simulink model "task8a_winkel"  (R2024a)
settings: Solver=VariableStepAuto  StartTime=0.0  StopTime=1.5  RelTol=1e-3
libraries: robotmaniplib x1, robotcorelib x1
settings Model: Creator=Nico  LastModifiedBy=laith
settings RTWCC: GPUComputeCapability=3.5

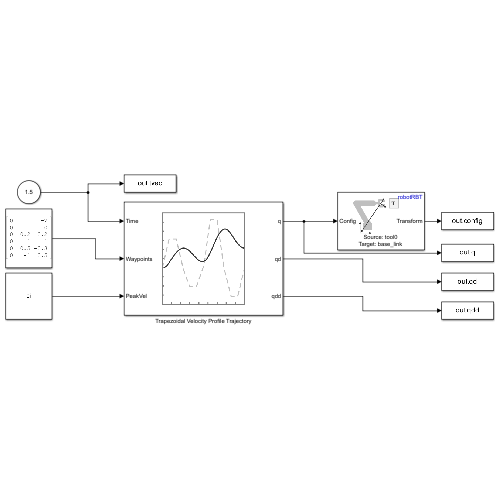
[thumbnail: Simulink's stored preview of the top-level diagram]
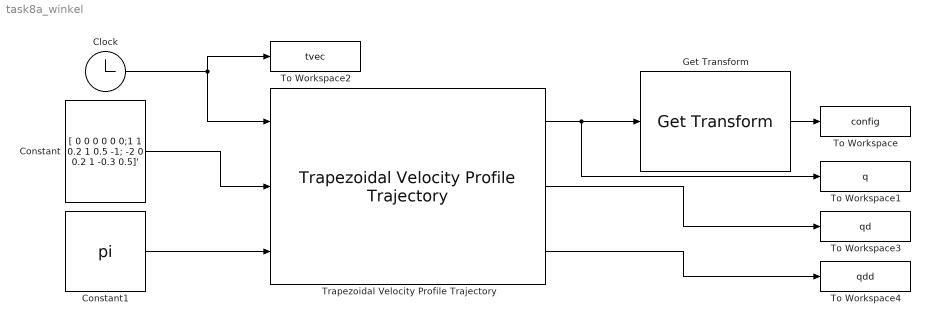
== system task8a_winkel ==
  Clock : Clock
      settings: Decimation=100
  Constant : Constant  Value="[ 0 0 0 0 0 0;1   1  0.2   1    0.5     -1;  -2  0  0.2   1 -0.3    0.5]'"
  Constant1 : Constant  Value=pi
  Get Transform : robotmaniplib/Get Transform  RigidBodyTree=robotRBT  SourceBody=tool0  TargetBody=base_link  SimulateUsing=Interpreted execution
  To Workspace : ToWorkspace  VariableName=config  SampleTime=-1
  To Workspace1 : ToWorkspace  VariableName=q  SampleTime=-1
      settings: Save2DSignal=2-D array (concatenate along first dimension)
  To Workspace2 : ToWorkspace  VariableName=tvec  SampleTime=-1
  To Workspace3 : ToWorkspace  VariableName=qd  SampleTime=-1
      settings: Save2DSignal=2-D array (concatenate along first dimension)
  To Workspace4 : ToWorkspace  VariableName=qdd  SampleTime=-1
      settings: Save2DSignal=2-D array (concatenate along first dimension)
  Trapezoidal Velocity Profile Trajectory : robotcorelib/Trapezoidal Velocity Profile Trajectory  WaypointSource=External  Waypoints=[ 0, -0.5, -1; 0, 0.5, 1 ]  NumParams=1  Parameter1=Peak Velocity  Parameter2=Acceleration  ParameterSource=External  PeakVelocity=[ 2; 2 ]  Acceleration=[ 1; 2 ]  EndTime=[ 1; 1 ]  AccelTime=[ 1; 2 ]  SimulateUsing=Interpreted execution
  wires:
  Constant/1 -> Trapezoidal Velocity Profile Trajectory/2
  Constant1/1 -> Trapezoidal Velocity Profile Trajectory/3
  Clock/1 -> Trapezoidal Velocity Profile Trajectory/1, To Workspace2/1
  Trapezoidal Velocity Profile Trajectory/1 -> To Workspace1/1, Get Transform/1
  Get Transform/1 -> To Workspace/1
  Trapezoidal Velocity Profile Trajectory/2 -> To Workspace3/1
  Trapezoidal Velocity Profile Trajectory/3 -> To Workspace4/1
